simulink model "reaction_pendulum"  (R2021b)
settings: Solver=FixedStepDiscrete  StartTime=0.0  StopTime=40  FixedStep=h  RelTol=1e-3  EnableMultiTasking=on
PreLoadFcn:
  | warning('off','MATLAB:dispatcher:InexactMatch');
InitFcn:
  | hwinit
settings Model: SimulationMode=external  ExtModeTrigDuration=100000  Creator=user  LastModifiedBy=jhines
settings SolverCC: AlgebraicLoopSolver=TrustRegion
settings DataIOCC: SaveFormat=Array  SignalLoggingSaveFormat=ModelDataLogs  SaveOutput=off  SignalLogging=off  DSMLogging=off  SaveTime=off  ReturnWorkspaceOutputs=off
settings OptimizationCC: ExpressionDepthLimit=2147483647  LifeSpan=inf
settings DebuggingCC: UnderspecifiedInitializationDetection=Classic  MergeDetectMultiDrivingBlocksExec=none  SolverPrmCheckMsg=warning  FcnCallInpInsideContextMsg=warning  StateNameClashWarn=warning  SFUnexpectedBacktrackingDiag=warning  SFNoUnconditionalDefaultTransitionDiag=warning  SFExecutionAtInitializationDiag=none  SFMachineParentedDataDiag=warning  ArithmeticOperatorsInVariantConditions=warning
settings HardwareCC: ProdBitPerPointer=32  ProdBitPerSizeT=32  ProdBitPerPtrDiffT=32  ProdLargestAtomicFloat=None  ProdIntDivRoundTo=Undefined  ProdEndianess=Unspecified  ProdWordSize=32  ProdHWDeviceType=32-bit Generic
settings ModelReferenceCC: PropagateSignalLabelsOutOfModel=off
settings SFSimCC: SimUseLocalCustomCode=off  CustomCodeUndefinedFunction=UseInterfaceOnly
settings RTWCC: Description=rpend RTDAC/USB2 (Visual C/C++)  SystemTargetFile=rtcon_rpend_usb2.tlc  TemplateMakefile=rtcon_rpend_vc_usb2_x64.tmf  RTWUseLocalCustomCode=off
settings CodeAppCC: StateflowObjectComments=on
settings STFCustomTargetCC: ModelReferenceCompliant=off  CombineOutputUpdateFcns=on  MatFileLogging=on  GRTInterface=off  SystemTargetFile=rtcon_rpend_usb2.tlc
settings GRTTargetCC: TargetLangStandard=C89/C90 (ANSI)  ModelReferenceCompliant=off  ParMdlRefBuildCompliant=off  CompOptLevelCompliant=off  ConcurrentExecutionCompliant=off  CPPClassGenCompliant=off  UseToolchainInfoCompliant=off  ExtMode=on  ExtModeMexFile=rtcon_ext_comm
settings ConfigComp: CovMetricSettings=dw  CovSaveCumulativeToWorkspaceVar=on  CovSaveSingleToWorkspaceVar=on  CovExternalEMLEnable=off  CovSFcnEnable=off

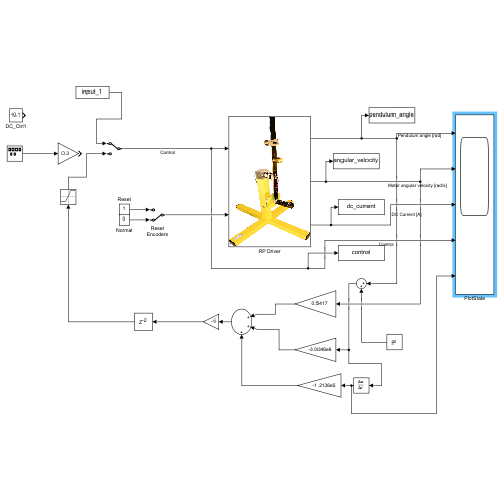
[thumbnail: Simulink's stored preview of the top-level diagram]
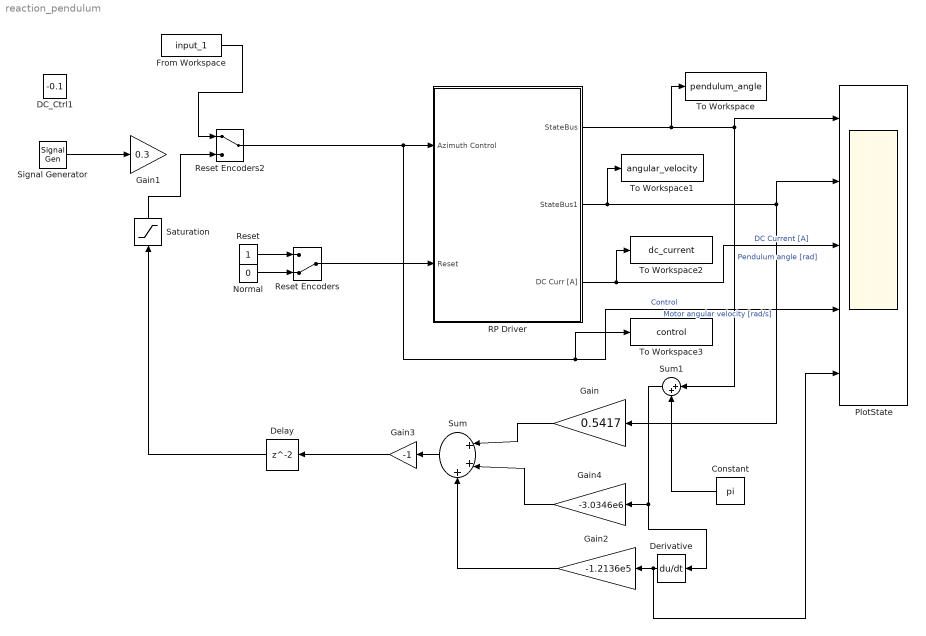
== system reaction_pendulum ==
  Constant : Constant  Value=pi
  DC_Ctrl1 : Constant  Value=-0.1
  Delay : Delay
  Derivative : Derivative
  From Workspace : FromWorkspace  VariableName=input_1
  Gain : Gain  Gain=0.5417
  Gain1 : Gain  Gain=0.3
  Gain2 : Gain  Gain=-1.2136e5
  Gain3 : Gain  Gain=-1
  Gain4 : Gain  Gain=-3.0346e6
  Normal : Constant  Value=0
  PlotState : Scope  NumInputPorts=5
  RP Driver : Subsystem
      mask Display: image(imread('rwp.JPG'))
  Reset : Constant
  Reset Encoders : ManualSwitch  CurrentSetting=0
  Reset Encoders2 : ManualSwitch
  Saturation : Saturate  UpperLimit=0.8  LowerLimit=-0.8
  Signal Generator : SignalGenerator  Frequency=1/2
  Sum : Sum  Inputs=|+++
  Sum1 : Sum  Inputs=|++
  To Workspace : ToWorkspace  VariableName=pendulum_angle  SaveFormat=Timeseries  SampleTime=-1
  To Workspace1 : ToWorkspace  VariableName=angular_velocity  SaveFormat=Timeseries  SampleTime=-1
  To Workspace2 : ToWorkspace  VariableName=dc_current  SaveFormat=Timeseries  SampleTime=-1
  To Workspace3 : ToWorkspace  VariableName=control  SaveFormat=Timeseries  SampleTime=-1
  wires:
  Normal/1 -> Reset Encoders/2
  Reset/1 -> Reset Encoders/1
  Reset Encoders/1 -> RP Driver/2(Reset)
  RP Driver/3(DC Curr [A]) -> To Workspace2/1, PlotState/3  "DC Current [A]"
  Reset Encoders2/1 -> To Workspace3/1, PlotState/4, RP Driver/1(Azimuth Control)  "Control"
  Signal Generator/1 -> Gain1/1
  RP Driver/2(StateBus1) -> To Workspace1/1, Gain/1, PlotState/2  "Motor angular velocity [rad/s]"
  RP Driver/1(StateBus) -> To Workspace/1, Sum1/1, PlotState/1  "Pendulum angle [rad]"
  Gain/1 -> Sum/1
  Gain2/1 -> Sum/3
  Sum/1 -> Gain3/1
  Gain3/1 -> Delay/1
  Delay/1 -> Saturation/1
  Derivative/1 -> PlotState/5, Gain2/1
  Saturation/1 -> Reset Encoders2/2
  Gain4/1 -> Sum/2
  Sum1/1 -> Gain4/1, Derivative/1
  Constant/1 -> Sum1/2
  From Workspace/1 -> Reset Encoders2/1

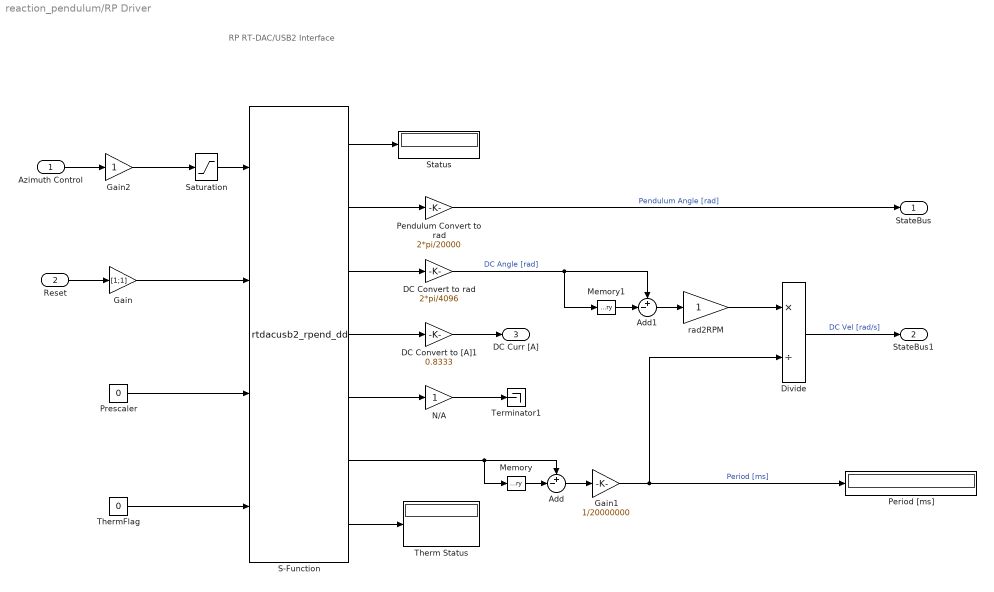
== system reaction_pendulum/RP Driver ==
  note: RP RT-DAC/USB2
      | Interface
  Azimuth Control : Inport
  Reset : Inport  Port=2
  Add : Sum  Inputs=+-|
  Add1 : Sum  Inputs=+-|
  DC Convert to [A]1 : Gain  Gain=0.8333  SaturateOnIntegerOverflow=on  OutDataTypeStr=Inherit: Same as input  ParamDataTypeStr=Inherit: Same as input
  DC Convert to rad : Gain  Gain=2*pi/4096  SaturateOnIntegerOverflow=on  OutDataTypeStr=Inherit: Same as input  ParamDataTypeStr=Inherit: Same as input
  Divide : Product  Inputs=*/
  Gain : Gain  Gain=[1;1]
  Gain1 : Gain  Gain=1/20000000
  Gain2 : Gain
  Memory : Memory
  Memory1 : Memory
  N/A : Gain  SaturateOnIntegerOverflow=on  OutDataTypeStr=Inherit: Same as input  ParamDataTypeStr=Inherit: Same as input
  Pendulum Convert to rad : Gain  Gain=2*pi/20000  SaturateOnIntegerOverflow=on  OutDataTypeStr=Inherit: Same as input  ParamDataTypeStr=Inherit: Same as input
  Period [ms] : Display
  Prescaler : Constant  Value=0
  S-Function : S-Function  FunctionName=rtdacusb2_rpend_dd  Parameters=1, h  SFunctionDeploymentMode=off  EnableBusSupport=off
  Saturation : Saturate  UpperLimit=1  LowerLimit=-1
  Status : Display
  Terminator1 : Terminator
  Therm Status : Display
  ThermFlag : Constant  Value=0
  rad2RPM : Gain  SaturateOnIntegerOverflow=on  OutDataTypeStr=Inherit: Same as input  ParamDataTypeStr=Inherit: Same as input
  StateBus : Outport  VectorParamsAs1DForOutWhenUnconnected=off
  StateBus1 : Outport  Port=2  VectorParamsAs1DForOutWhenUnconnected=off
  DC Curr [A] : Outport  Port=3  VectorParamsAs1DForOutWhenUnconnected=off
  wires:
  S-Function/7 -> Therm Status/1
  S-Function/5 -> N/A/1
  S-Function/4 -> DC Convert to [A]1/1
  ThermFlag/1 -> S-Function/4
  Prescaler/1 -> S-Function/3
  Gain/1 -> S-Function/2
  DC Convert to [A]1/1 -> DC Curr [A]/1
  Divide/1 -> StateBus1/1  "DC Vel [rad/s]"
  rad2RPM/1 -> Divide/1
  Add1/1 -> rad2RPM/1
  Memory1/1 -> Add1/2
  N/A/1 -> Terminator1/1
  S-Function/6 -> Add/1, Memory/1
  Gain2/1 -> Saturation/1
  Gain1/1 -> Period [ms]/1, Divide/2  "Period [ms]"
  Add/1 -> Gain1/1
  Memory/1 -> Add/2
  DC Convert to rad/1 -> Add1/1, Memory1/1  "DC Angle [rad]"
  S-Function/3 -> DC Convert to rad/1
  Pendulum Convert to rad/1 -> StateBus/1  "Pendulum Angle [rad]"
  S-Function/2 -> Pendulum Convert to rad/1
  S-Function/1 -> Status/1
  Saturation/1 -> S-Function/1
  Reset/1 -> Gain/1
  Azimuth Control/1 -> Gain2/1
